simulink model "Project"  (R2025a)
settings: Solver=VariableStepAuto  StartTime=0.0  StopTime=10.0  RelTol=1e-3
libraries: dspfdesign x5, simulink x5, dspsnks4 x1, dspvision x1
settings Model: Creator=G3NZ  LastModifiedBy=G3NZ

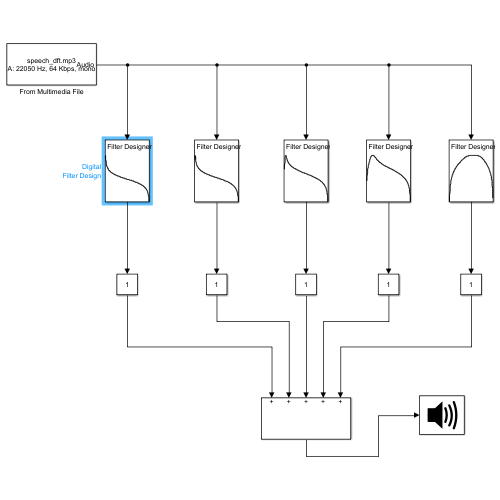
[thumbnail: Simulink's stored preview of the top-level diagram]
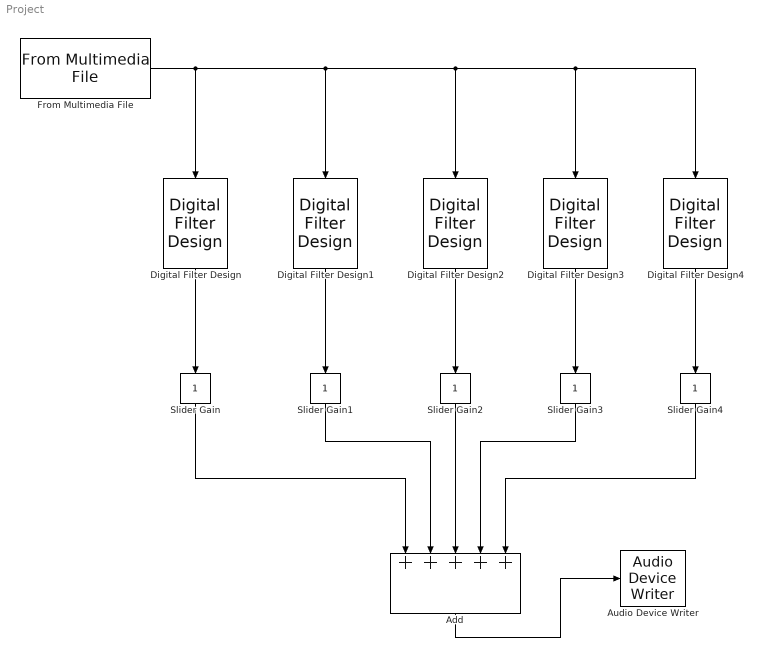
== system Project ==
  Add : Sum  Inputs=+++++
  Audio Device Writer : dspsnks4/Audio Device Writer  Driver=DirectSound  Device=Default  InheritSampleRate=on  SampleRate=44100  BitDepth=16-bit integer  BufferSize=4096  NumBuffers=10  DefaultOutputChannelMapping=on  OutputChannelMapping=1:2  OutputNumUnderrunSamples=off  DriverIdx=1  DeviceWarnFlag=''
  Digital Filter Design{,1..4} (5 alike) : dspfdesign/Digital Filter Design  mwdsp_browser_bugfix_var=off
  From Multimedia File : dspvision/From Multimedia File  inputFilename=C:\Program Files\MATLAB\R2025a\toolbox\dsp\dsp\samples\speech_dft.mp3  readRange=[1 Inf]  loop=on  numPlays=inf  outputStreams=Audio only  videoDataType=single  audioDataType=double  inheritSampleTime=on  userDefinedSampleTime=1/30  noAudioOutput=off  isIntensityVideo=off  fourcc=RGB  colorVideoFormat=One multidimensional signal  outputEOF=off  dataOrg=Column-major  audioFrameSize=1024  computeAudioFrameSize=off  outSamplingMode=Sample based
      settings: LibrarySourceBlock=dspsrcs4/From Multimedia File
  Slider Gain{,1..4} (5 alike) : simulink/Math Operations/Slider Gain  gain=1  low=0.251  high=3.981
  wires:
  Digital Filter Design/1 -> Slider Gain/1
  Digital Filter Design1/1 -> Slider Gain1/1
  Digital Filter Design2/1 -> Slider Gain2/1
  Digital Filter Design3/1 -> Slider Gain3/1
  Digital Filter Design4/1 -> Slider Gain4/1
  Slider Gain/1 -> Add/1
  Slider Gain1/1 -> Add/2
  Slider Gain2/1 -> Add/3
  Slider Gain3/1 -> Add/4
  Slider Gain4/1 -> Add/5
  Add/1 -> Audio Device Writer/1
  From Multimedia File/1 -> Digital Filter Design1/1, Digital Filter Design4/1, Digital Filter Design3/1, Digital Filter Design2/1, Digital Filter Design/1
